simulink model "may7bdrc"  (Simulink 8.5)
settings: Solver=ode4  StartTime=0.0  StopTime=inf  FixedStep=BKIN_STEP_TIME  RelTol=1e-3
model workspace (MAT data in the model file):
  BARRIER_ROW = 5
  BKIN_KINEMATIC_FRAME_SIZE = 400
  BKIN_STEP_TIME = 0.00025
  CIRCLE_ROW = 2
  CIRCLE_STROKE = 10
  CIRCLE_STROKE_W = 11
  E_BARRIER_HIT = 6
  E_COLLISION_HIT = 7
  E_ENTER_PRESHOT_AREA = 2
  E_ENTER_START_AREA = 12
  E_EXIT = 13
  E_EXIT_PRESHOT_AREA = 10
  E_GOAL_HIT = 8
  E_GOAL_REACHED = 5
  E_NO_EVENT = 0
  E_PRESHOT_ROW = 4
  E_TARGET_OUT_OF_BOUNDS = 9
  E_TRIAL_BEGIN = 1
  E_TRIAL_ENDED = 3
  FIRST_STATE_FILL = 9
  FORCE_MULTIPLIER = 1
  F_BUMP = 1
  GOAL_ROW = 8
  GOAL_TIME = 15
  HEIGHT = 6
  INVISIBLE_FILL = 15
  LOAD_ROW = 4
  MASS_BARRIER = 6
  MASS_CIRCLE = 2
  MASS_RECT = 3
  NEW_FLOAT = 10
  NEW_ROW = 9
  NEW_TEXTSIZE = 11
  PERT_DUR = 5
  PERT_RAMP = 4
  PRESHOT_ROW = 7
  RADIUS_LOG = 4
  RADIUS_VIS = 5
  RECT_FILL = 12
  RECT_ROW = 3
  RECT_STROKE = 13
  RECT_STROKE_W = 14
  ROTATION = 7
  SECONDS = 1
  SECOND_STATE_FILL = 8
  SHOT_READY_TIME = 13
  SHOT_SET_TIME = 14
  START_HOLD_TIME = 12
  START_ROW = 6
  TRIAL_FAILURE = 11
  WIDTH = 3
  col_x = 1
  col_y = 2
StartFcn:
  |  warndlg('Dexterit-E models cannot run under simulation. Please compile your model and run it from within Dexterit-E.');set_param(bdroot,'SimulationCommand','stop')
undefined symbols (not defined in the file): slselsubs
libraries: Video x7, General x3, KINARM_loads x2, KINARM_EP_loads x1, KINARM_general x1, simulink x1, slrtlib x1
(part 1 of 3)
settings Model: Creator=Chris Grebeldinger  LastModifiedBy=User  ModifiedComment=chris -- Wed Feb 16 09:18:30 2005 -- Version 1.1384  ModifiedHistory=Feb 16/05 - Add error repeat, add offset ramp  ExtModeArmWhenConnect=off  ExtModeLogAll=off
settings SolverCC: AutoInsertRateTranBlk=on
settings DataIOCC: LimitDataPoints=off  SaveOutput=off  SaveTime=off  SignalLoggingName=sigsOut
settings OptimizationCC: BlockReduction=off  BooleanDataType=off  OptimizeBlockIOStorage=off  BufferReuse=off  GlobalBufferReuse=off  ExpressionFolding=off  LocalBlockOutputs=off  InitFltsAndDblsToZero=on
settings DebuggingCC: SaveWithParameterizedLinksMsg=none  SignalResolutionControl=TryResolveAllWithWarning  MultiTaskDSMMsg=warning  FcnCallInpInsideContextMsg=EnableAllAsWarning  BusObjectLabelMismatch=none  StrictBusMsg=ErrorOnBusTreatedAsVector
settings HardwareCC: ProdIntDivRoundTo=Zero  ProdEndianess=LittleEndian  ProdLongLongMode=on  ProdHWDeviceType=Generic->32-bit x86 compatible  TargetHWDeviceType=32-bit Generic
settings SFSimCC: SimParseCustomCode=off
settings RTWCC: Description=Simulink Real-Time  SystemTargetFile=slrt.tlc  TemplateMakefile=slrt_default_tmf  CodeExecutionProfiling=on  RTWCompilerOptimization=on
settings CodeAppCC: MaxIdLength=63
settings SimulinkRealTimeCC: TargetFcnLib=ansi_tfl_tmw.mat  GeneratePreprocessorConditionals=Disable all

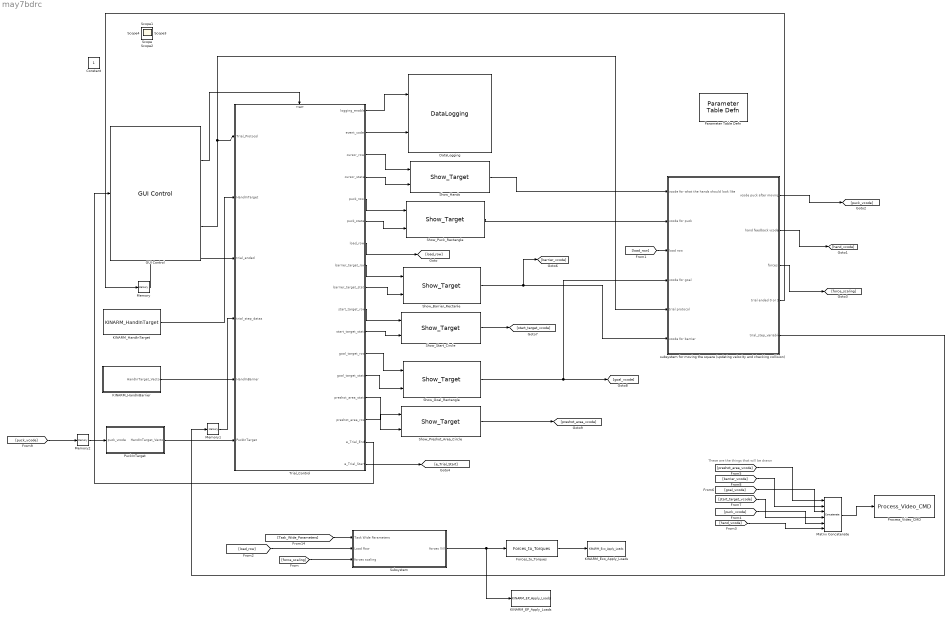
== system may7bdrc ==
  note: These are the things that will be drawn
  DataLogging : General/DataLogging  log_event_codes=on  log_analog_inputs=off  show_time_remaining=off  ecat_include=on
  Forces_to_Torques : KINARM_loads/Forces_to_Torques
  GUI Control : General/GUI Control  task_version=1.0  show_repeat_trial_flag=off  use_custom_tp=off  target_type_str=Circle  Target_Type=1  XYcols=[1 2]  Vcols=3  Lcols=4  indices_padding=[0 0 0 0;0 0 0 0]  target_table_rows=64  load_table_rows=20  tp_table_rows=100
  KINARM_EP_Apply_Loads : KINARM_EP_loads/KINARM_EP_Apply_Loads  up_duration=1500  down_duration=1500  max_force=20
  KINARM_Exo_Apply_Loads : KINARM_loads/KINARM_Exo_Apply_Loads  up_duration=1500  down_duration=1500  max_torque=5  limit_motors=off
  KINARM_HandInBarrier : Subsystem  AncestorBlock=KINARM_general/KINARM_HandInTarget  mask(KINARM_HandInTarget){use_dominant_hand=on, target_type=Rectangle, num_states=1, attribcol1=[WIDTH HEIGHT ROTATION], attribcol2=[0 0 0], attribcol3=[0 0 0], attribcol4=[0 0 0], attribcol5=[0 0 0]}
      mask prompts: use_dominant_hand "Use "arm to be assessed"?"; target_type "Type of Target"; num_states "Number of Target States"; attribcol1 "State 1 Target Table Column(s)"; attribcol2 "State 2 Target Table Column(s)"; attribcol3 "State 3 Target Table Column(s)"; attribcol4 "State 4 Target Table Column(s)"; attribcol5 "State 5 Target Table Column(s)"
      mask help: This block returns a vector or array corresponding to the Target_Table rows indicating whether the specified hand is in (=1) or out (=0) of each of the targets.
      mask init:
      | block_path = gcb;  % store block path, as gcb may change with block operations
      | 
      | %%% Get the model's workspace, because it is required to evaluate constants from the Parameter Table Def'n block
      | modelName=bdroot(block_path);
      | modelWorkspace = get_param(modelName, 'ModelWorkspace');
      | 
      | %%% Handle background colours if link status changes.  
      | checkBackgroundColour(block_path, 'KINARM_general');
      | 
      | %%% create the names of the input and output ports to display on the mask
      | % Select only the desired states for output. The output port is also renamed to reflect 
      | % whether the output is a vector (in the case of a single state) or an array (of vectors, 
      | % one for each of multiple states).
      | 
      | numStates = str2double( get_param(block_path, 'num_states') );
      | 
      | if numStates == 1
      | 	set_param([block_path '/Selected States'], 'Value', '[1]');
      | 	outputname = 'HandInTarget_Vector';
      | elseif numStates == 2
      | 	set_param([block_path '/Selected States'], 'Value', '[1,2]');
      | 	outputname = 'HandInTarget_Array';
      | elseif numStates == 3
      | 	set_param([block_path '/Selected States'], 'Value', '[1,2,3]');
      | 	outputname = 'HandInTarget_Array';
      | elseif numStates == 4
      | 	set_param([block_path '/Selected States'], 'Value', '[1,2,3,4]');
      | 	outputname = 'HandInTarget_Array';
      | else
      | 	set_param([block_path '/Selected States'], 'Value', '[1,2,3,4,5]');
      | 	outputname = 'HandInTarget_Array';
      | end
      | output_block=char(find_system(gcb,'LookUnderMasks','all','FollowLinks','on','SearchDepth',1,'BlockType','Outport'));
      | set_param(output_block, 'Name', outputname);
      | 
      | 
      | %%%%%%%%%%%%%%%%%%%%%%%%%%%%%%%%%%%%%%%%%%%%%%%%%%%%%%%%%%%%%
      | %%% Check and format the input strings for the vectors of column entires
      | targetTypeStr=get_param(block_path, 'target_type');
      | 
      | switch targetTypeStr(1:3)
      | 	case 'Cir',		numCol = 1;
      | 	case 'Ell',		numCol = 3;
      |     case 'Rec',		numCol = 3;
      |     case 'Lin',		numCol = 3;
      |     case 'Tri',		numCol = 4;
      | 	otherwise,		numCol = 1;
      | end
      | 
      | for ii = 1:numStates
      | 	variableName = ['attribcol' num2str(ii)];
      | 	attribcoltext = get_param(block_path, variableName);
      | 	attribcoltext = checkUserInputVectorLength(attribcoltext, numCol);
      | 	set_param(block_path, variableName, attribcoltext);
      | end
      | 
      | for ii = 1+numStates:5
      | 	variableName = ['attribcol' num2str(ii)];
      |     if numCol == 1
      |         outstr = '[0]';
      |     else
      |         outstr = mat2str(zeros(1, numCol));
      |     end
      |     set_param(block_path, variableName, outstr);
      | end
      | 
      | %%%%%%%%%%%%%%%%%%%%%%%%%%%%%%%%%%%%%%%%%%%%%%%%%%%%%%%%%%%%%
      | %%% Create the text to show on the mask
      | numStates = str2num(get_param(block_path, 'num_states'));
      | columntext='(columns: ';
      | 
      | for ii = 1:numStates
      | 	variableName = ['attribcol' num2str(ii)];
      | 	attribcolString = get_param(block_path, variableName);
      | 	if isempty(modelWorkspace)
      | 		% if the block is part of a library, then modelWorkspace will be empty and the other code to evaluate attribcolStringEval will fail
      | 		attribcolStringEval = '3';
      | 	else
      | 		[attribcolValue, errorMessage] = BKINevalin(modelWorkspace, attribcolString);
      | 		attribcolStringEval = mat2str( attribcolValue );
      | 	end
      | 	if ii > 1
      | 		columntext = [columntext, '; ', attribcolStringEval];
      | 	else
      | 		columntext = [columntext, attribcolStringEval];
      | 	end
      | end
      | 
      | % Add formatting spaces so that the mask looks nice
      | columntext=strvcat([columntext ')'],' ', ' ');
      mask Help:
      | Used to determine if the hand (fingertip) is in any of the targets in the Target_Table.
      | <P>
      | <B><I>Use of this block requires that the DataLogging block (General library) be set to log KINARM data.</I></B>
      | 
      | <H2>Library </H2>
      | KINARM general
      | 
      | <H2>Description </H2>
      | This block returns a vector or array corresponding to the Target_Table rows indicating whether the specified hand (i.e. fingertip) is in or out of each of the targets.  Each element in the output vector or output array will be either a 0 (hand not in target) or a 1 (hand in target).
      | <P>
      | A vector is returned if only one target state is specified in each target row (see Parameters and Dialog Box), with each index of the vector corresponding to a row in the target table.  An array is returned if more than one target state is specified in a target row, with each row of the array corresponding to a target row and each column corresponding to the nth target state specified in each target row.
      | <P>
      | The output vector or array is typically used by a stateflow chart to affect behavior of the system.  Because this block returns hand-in-target information for all targets in the target table, multiple targets can be monitored at once (i.e. the Stateflow chart could have certain transitions that occur if the hand is in one target and other transitions if it is in a different target).  Likewise, because this block returns hand-in-target information for multiple states of a single target, those multiple states can be monitored simultaneously.
      | <P>
      | Because the KINARM_HandInTarget block returns information for only one hand, two copies of this block are required if information for both hands is desired.
      | <P>
      | 
      | <H2>Parameters and Dialog Box</H2>
      | <B>Use "arm to be assessed"?:</B> this checkbox determines which hand is used by this block. In Dexterit-E the operator selects the "arm to be assessed" using radio buttons.
      | When this box is checked the output of this block is derived from the hand information corresponding to the arm selection made by the operator in Dexterit-E.
      | When this box is unchecked the output of this block is derived from the contralateral arm.
      | (Note: to obtain information about both hands, then 2 separate copies of this block are required - one for each hand.)
      | <P>
      | <B>Type of Target:</B> Enter the type of target specified in the target table:
      | <P>
      | <B>Number of Target States:</B> Enter the number of target states specified in each target row.  Up to four target states are allowed per target row.
      | <P>
      | <B>State <n> Target Table Columns:</B> Enter the columns in the Target Table that specify the relevant target attributes.  Do this for each target state.
      | For a circle, enter the columns corresponding to logical radius (e.g. 4)
      | <BR>For an ellipse, enter the columns corresponding to major radius, minor radius, rotation angle (e.g. [4, 5, 6]).
      | <BR>For a rectangle, enter the columns corresponding to length, height, and rotation angle (e.g. [4, 5, 6]).
      | <BR>For a line, enter the columns corresponding to stroke width, endpoint in x, and endpoint in y (e.g. [3, 4, 5]).
      | <BR>For a triangle, enter the columns corresponding to length, height, peak offset, and rotation angle (e.g. [4, 5, 6, 7]).
      | 
      | <H2>Examples</H2>
      | <B>Example 1.</B>  Suppose a target row will be used to define 1 state for a circle type target and the radius of the visual target is the same radius to be used for determination of hand-in-target.  The related Target Table column is: column 6 = radius.  For this example, "State 1 Target Table Columns" would equal [6].
      | <P>
      | 
      | <B>Example 2.</B>  Suppose a target row will be used to define 1 state for a circle type target, but the radius of the visual target will be different than the radius to be used for determination of hand-in-target.  This option allows independent control over the size of the visual target versus the accuracy needed to be considered "in the target".  The related Target Table columns are: column 6 = radius1 (i.e. radius to target to be drawn); column 7 = radius2 (i.e. radius to be used for hand-in-target) .  For this example, "State 1 Target Table Columns" would equal [7].
      | <P>
      | <B>Example 3.</B>  Suppose a target row will be used to define 2 states for a circle type target, where the radius of the visual target will be a constant, but depending on the state of the system, one of 2 other and different radii will be used for determination of hand-in-target.  The related Target Table columns are: column 6 = radius1 (i.e. radius to target to be drawn); column 7 = radius2 (i.e. radius to be used for hand-in-target for state 1); column 8 = radius3 (i.e. radius to be used for hand-in-target for state 2).  For this example, "State 1 Target Table Columns" would equal [7], while "State 2 Target Table Columns" would equal [8].
      | <P>
      | 
      | <H2>Related Blocks </H2>
      | DataLogging
      mask TypeOptions target_type: Circle | Ellipse | Rectangle | Line | Triangle
      mask Callback target_type:
      | %%%%
      | % Because of bugs iN R2007, R2010a and R2013a (which have been reported to Mathworks), the following code
      | % is required here because in the Initialization Section it will ONLY correctly update those Mask Parameters that are hidden
      | % when the OK button is clicked (NOTE: the initialization code will correctly update all Mask Parameters when the Apply button
      | % is clicked, the bug is that it should also update everything when the OK button is clicked in the absence of an Apply click)
      | %
      | % Adding a set_param call which updates one of the mask parameters will call the initialization code to run, which "avoids"
      | % this bug. This code should be removed once Mathworks has fixed this bug.
      | 
      | temp = get_param(gcb, 'target_type');
      | set_param(gcb, 'target_type', temp);
      mask TypeOptions num_states: 1 | 2 | 3 | 4 | 5
      mask Callback num_states:
      | num_states = str2num(get_param(gcb, 'num_states'));
      | vis = get_param(gcb, 'MaskVisibilities');
      | 
      | % Select only the desired states for output. The output port is also renamed to reflect
      | % whether the output is a vector (in the case of a single state) or an array (of vectors,
      | % one for each of multiple states).
      | output_block=char(find_system(gcb, 'LookUnderMasks', 'all', 'FollowLinks', 'on', 'SearchDepth', 1, 'BlockType', 'Outport'));
      | 
      | if num_states == 1
      | % % % 	set_param([gcb '/Selected States'], 'Value', '[1]');
      | % % % 	set_param(output_block, 'Name', 'HandInTarget_Vector');
      | 	vis{5} = 'off';
      | 	vis{6} = 'off';
      | 	vis{7} = 'off';
      | 	vis{8} = 'off';
      | elseif num_states == 2
      | % % % 	set_param([gcb '/Selected States'], 'Value', '[1,2]');
      | % % % 	set_param(output_block, 'Name', 'HandInTarget_Array');
      | 	vis{5} = 'on';
      | 	vis{6} = 'off';
      | 	vis{7} = 'off';
      | 	vis{8} = 'off';
      | elseif num_states == 3
      | % % % 	set_param([gcb '/Selected States'], 'Value', '[1,2,3]');
      | % % % 	set_param(output_block, 'Name','HandInTarget_Array');
      | 	vis{5} = 'on';
      | 	vis{6} = 'on';
      | 	vis{7} = 'off';
      | 	vis{8} = 'off';
      | elseif num_states == 4
      | % % % 	set_param([gcb '/Selected States'], 'Value', '[1,2,3,4]');
      | % % % 	set_param(output_block, 'Name','HandInTarget_Array');
      | 	vis{5} = 'on';
      | 	vis{6} = 'on';
      | 	vis{7} = 'on';
      | 	vis{8} = 'off';
      | else
      | % % % 	set_param([gcb '/Selected States'], 'Value', '[1,2,3,4,5]');
      | % % % 	set_param(output_block, 'Name', 'HandInTarget_Array');
      | 	vis{5} = 'on';
      | 	vis{6} = 'on';
      | 	vis{7} = 'on';
      | 	vis{8} = 'on';
      | end
      | set_param(gcb, 'MaskVisibilities', vis);
      mask Display:
      | disp(columntext);
      | port_label('output',1,outputname);
  KINARM_HandInTarget : KINARM_general/KINARM_HandInTarget  use_dominant_hand=on  target_type=Circle  num_states=1  attribcol1=[RADIUS_LOG]  attribcol2=[0]  attribcol3=[0]  attribcol4=[0]  attribcol5=[0]
  Matrix Concatenate : Concatenate  NumInputs=6  Mode=Multidimensional array
  Memory : Memory
  Memory1 : Memory
  Memory2 : Memory
  Parameter Table Defn : General/Parameter Table Defn  ShowInLibBrowser=0
  Process_Video_CMD : Video/Process_Video_CMD  video_delay=0
  PuckInTarget : Subsystem  AncestorBlock=KINARM_general/KINARM_HandInTarget  mask(KINARM_HandInTarget){use_dominant_hand=on, target_type=Rectangle, num_states=1, attribcol1=[WIDTH HEIGHT ROTATION], attribcol2=[0 0 0], attribcol3=[0 0 0], attribcol4=[0 0 0], attribcol5=[0 0 0]}
      mask prompts: use_dominant_hand "Use "arm to be assessed"?"; target_type "Type of Target"; num_states "Number of Target States"; attribcol1 "State 1 Target Table Column(s)"; attribcol2 "State 2 Target Table Column(s)"; attribcol3 "State 3 Target Table Column(s)"; attribcol4 "State 4 Target Table Column(s)"; attribcol5 "State 5 Target Table Column(s)"
      mask help: This block returns a vector or array corresponding to the Target_Table rows indicating whether the specified hand is in (=1) or out (=0) of each of the targets.
      mask init: same as may7bdrc/KINARM_HandInBarrier
      mask Help:
      | Used to determine if the hand (fingertip) is in any of the targets in the Target_Table.
      | <P>
      | <B><I>Use of this block requires that the DataLogging block (General library) be set to log KINARM data.</I></B>
      | 
      | <H2>Library </H2>
      | KINARM general
      | 
      | <H2>Description </H2>
      | This block returns a vector or array corresponding to the Target_Table rows indicating whether the specified hand (i.e. fingertip) is in or out of each of the targets.  Each element in the output vector or output array will be either a 0 (hand not in target) or a 1 (hand in target).
      | <P>
      | A vector is returned if only one target state is specified in each target row (see Parameters and Dialog Box), with each index of the vector corresponding to a row in the target table.  An array is returned if more than one target state is specified in a target row, with each row of the array corresponding to a target row and each column corresponding to the nth target state specified in each target row.
      | <P>
      | The output vector or array is typically used by a stateflow chart to affect behavior of the system.  Because this block returns hand-in-target information for all targets in the target table, multiple targets can be monitored at once (i.e. the Stateflow chart could have certain transitions that occur if the hand is in one target and other transitions if it is in a different target).  Likewise, because this block returns hand-in-target information for multiple states of a single target, those multiple states can be monitored simultaneously.
      | <P>
      | Because the KINARM_HandInTarget block returns information for only one hand, two copies of this block are required if information for both hands is desired.
      | <P>
      | 
      | <H2>Parameters and Dialog Box</H2>
      | <B>Use "arm to be assessed"?:</B> this checkbox determines which hand is used by this block. In Dexterit-E the operator selects the "arm to be assessed" using radio buttons.
      | When this box is checked the output of this block is derived from the hand information corresponding to the arm selection made by the operator in Dexterit-E.
      | When this box is unchecked the output of this block is derived from the contralateral arm.
      | (Note: to obtain information about both hands, then 2 separate copies of this block are required - one for each hand.)
      | <P>
      | <B>Type of Target:</B> Enter the type of target specified in the target table:
      | <P>
      | <B>Number of Target States:</B> Enter the number of target states specified in each target row.  Up to four target states are allowed per target row.
      | <P>
      | <B>State <n> Target Table Columns:</B> Enter the columns in the Target Table that specify the relevant target attributes.  Do this for each target state.
      | For a circle, enter the columns corresponding to logical radius (e.g. 4)
      | <BR>For an ellipse, enter the columns corresponding to major radius, minor radius, rotation angle (e.g. [4, 5, 6]).
      | <BR>For a rectangle, enter the columns corresponding to length, height, and rotation angle (e.g. [4, 5, 6]).
      | <BR>For a line, enter the columns corresponding to stroke width, endpoint in x, and endpoint in y (e.g. [3, 4, 5]).
      | <BR>For a triangle, enter the columns corresponding to length, height, peak offset, and rotation angle (e.g. [4, 5, 6, 7]).
      | 
      | <H2>Examples</H2>
      | <B>Example 1.</B>  Suppose a target row will be used to define 1 state for a circle type target and the radius of the visual target is the same radius to be used for determination of hand-in-target.  The related Target Table column is: column 6 = radius.  For this example, "State 1 Target Table Columns" would equal [6].
      | <P>
      | 
      | <B>Example 2.</B>  Suppose a target row will be used to define 1 state for a circle type target, but the radius of the visual target will be different than the radius to be used for determination of hand-in-target.  This option allows independent control over the size of the visual target versus the accuracy needed to be considered "in the target".  The related Target Table columns are: column 6 = radius1 (i.e. radius to target to be drawn); column 7 = radius2 (i.e. radius to be used for hand-in-target) .  For this example, "State 1 Target Table Columns" would equal [7].
      | <P>
      | <B>Example 3.</B>  Suppose a target row will be used to define 2 states for a circle type target, where the radius of the visual target will be a constant, but depending on the state of the system, one of 2 other and different radii will be used for determination of hand-in-target.  The related Target Table columns are: column 6 = radius1 (i.e. radius to target to be drawn); column 7 = radius2 (i.e. radius to be used for hand-in-target for state 1); column 8 = radius3 (i.e. radius to be used for hand-in-target for state 2).  For this example, "State 1 Target Table Columns" would equal [7], while "State 2 Target Table Columns" would equal [8].
      | <P>
      | 
      | <H2>Related Blocks </H2>
      | DataLogging
      mask TypeOptions target_type: Circle | Ellipse | Rectangle | Line | Triangle
      mask Callback target_type:
      | %%%%
      | % Because of bugs iN R2007, R2010a and R2013a (which have been reported to Mathworks), the following code
      | % is required here because in the Initialization Section it will ONLY correctly update those Mask Parameters that are hidden
      | % when the OK button is clicked (NOTE: the initialization code will correctly update all Mask Parameters when the Apply button
      | % is clicked, the bug is that it should also update everything when the OK button is clicked in the absence of an Apply click)
      | %
      | % Adding a set_param call which updates one of the mask parameters will call the initialization code to run, which "avoids"
      | % this bug. This code should be removed once Mathworks has fixed this bug.
      | 
      | temp = get_param(gcb, 'target_type');
      | set_param(gcb, 'target_type', temp);
      mask TypeOptions num_states: 1 | 2 | 3 | 4 | 5
      mask Callback num_states:
      | num_states = str2num(get_param(gcb, 'num_states'));
      | vis = get_param(gcb, 'MaskVisibilities');
      | 
      | % Select only the desired states for output. The output port is also renamed to reflect
      | % whether the output is a vector (in the case of a single state) or an array (of vectors,
      | % one for each of multiple states).
      | output_block=char(find_system(gcb, 'LookUnderMasks', 'all', 'FollowLinks', 'on', 'SearchDepth', 1, 'BlockType', 'Outport'));
      | 
      | if num_states == 1
      | % % % 	set_param([gcb '/Selected States'], 'Value', '[1]');
      | % % % 	set_param(output_block, 'Name', 'HandInTarget_Vector');
      | 	vis{5} = 'off';
      | 	vis{6} = 'off';
      | 	vis{7} = 'off';
      | 	vis{8} = 'off';
      | elseif num_states == 2
      | % % % 	set_param([gcb '/Selected States'], 'Value', '[1,2]');
      | % % % 	set_param(output_block, 'Name', 'HandInTarget_Array');
      | 	vis{5} = 'on';
      | 	vis{6} = 'off';
      | 	vis{7} = 'off';
      | 	vis{8} = 'off';
      | elseif num_states == 3
      | % % % 	set_param([gcb '/Selected States'], 'Value', '[1,2,3]');
      | % % % 	set_param(output_block, 'Name','HandInTarget_Array');
      | 	vis{5} = 'on';
      | 	vis{6} = 'on';
      | 	vis{7} = 'off';
      | 	vis{8} = 'off';
      | elseif num_states == 4
      | % % % 	set_param([gcb '/Selected States'], 'Value', '[1,2,3,4]');
      | % % % 	set_param(output_block, 'Name','HandInTarget_Array');
      | 	vis{5} = 'on';
      | 	vis{6} = 'on';
      | 	vis{7} = 'on';
      | 	vis{8} = 'off';
      | else
      | % % % 	set_param([gcb '/Selected States'], 'Value', '[1,2,3,4,5]');
      | % % % 	set_param(output_block, 'Name', 'HandInTarget_Array');
      | 	vis{5} = 'on';
      | 	vis{6} = 'on';
      | 	vis{7} = 'on';
      | 	vis{8} = 'on';
      | end
      | set_param(gcb, 'MaskVisibilities', vis);
      mask Display:
      | disp(columntext);
      | port_label('output',1,outputname);
  Show_Barrier_Rectanle : Video/Show_Target  target_type=Rectangle  num_states=2  attribcol1=[FIRST_STATE_FILL RECT_STROKE RECT_STROKE_W WIDTH HEIGHT ROTATION]  attribcol2=[SECOND_STATE_FILL RECT_STROKE RECT_STROKE_W WIDTH HEIGHT ROTATION]  attribcol3=[0 0 0 0 0 0]  attribcol4=[0 0 0 0 0 0]  attribcol5=[0 0 0 0 0 0]  stateindices_padding=[0 0 0 0 0;0 0 0 0 0;0 0 0 0 0;0 0 0 0 0;0 0 0 0 0]  source=dialog  opacity=100  target_display=Both subject and operator displays  num_col=6
  Show_Goal_Rectangle : Video/Show_Target  target_type=Rectangle  num_states=3  attribcol1=[INVISIBLE_FILL RECT_STROKE RECT_STROKE_W WIDTH HEIGHT ROTATION]  attribcol2=[FIRST_STATE_FILL RECT_STROKE RECT_STROKE_W WIDTH HEIGHT ROTATION]  attribcol3=[SECOND_STATE_FILL RECT_STROKE RECT_STROKE_W WIDTH HEIGHT ROTATION]  attribcol4=[0 0 0 0 0 0]  attribcol5=[0 0 0 0 0 0]  stateindices_padding=[0 0 0 0 0;0 0 0 0 0;0 0 0 0 0;0 0 0 0 0;0 0 0 0 0]  source=dialog  opacity=100  target_display=Both subject and operator displays  num_col=6
  Show_Hands : Video/Show_Target  target_type=Circle  num_states=2  attribcol1=[FIRST_STATE_FILL CIRCLE_STROKE CIRCLE_STROKE_W WIDTH]  attribcol2=[SECOND_STATE_FILL CIRCLE_STROKE CIRCLE_STROKE_W WIDTH]  attribcol3=[0 0 0 0]  attribcol4=[0 0 0 0]  attribcol5=[0 0 0 0]  stateindices_padding=[0 0 0 0 0 0 0;0 0 0 0 0 0 0;0 0 0 0 0 0 0;0 0 0 0 0 0 0;0 0 0 0 0 0 0]  source=dialog  opacity=100  target_display=Both subject and operator displays  num_col=4
  Show_Preshot_Area_Circle : Video/Show_Target  target_type=Circle  num_states=3  attribcol1=[INVISIBLE_FILL CIRCLE_STROKE CIRCLE_STROKE_W WIDTH]  attribcol2=[FIRST_STATE_FILL CIRCLE_STROKE CIRCLE_STROKE_W WIDTH]  attribcol3=[SECOND_STATE_FILL CIRCLE_STROKE CIRCLE_STROKE_W WIDTH]  attribcol4=[0 0 0 0]  attribcol5=[0 0 0 0]  stateindices_padding=[0 0 0 0 0 0 0;0 0 0 0 0 0 0;0 0 0 0 0 0 0;0 0 0 0 0 0 0;0 0 0 0 0 0 0]  source=dialog  opacity=100  target_display=Both subject and operator displays  num_col=4
  Show_Puck_Rectangle : Video/Show_Target  target_type=Rectangle  num_states=3  attribcol1=[INVISIBLE_FILL RECT_STROKE RECT_STROKE_W WIDTH HEIGHT ROTATION]  attribcol2=[FIRST_STATE_FILL RECT_STROKE RECT_STROKE_W WIDTH HEIGHT ROTATION]  attribcol3=[SECOND_STATE_FILL RECT_STROKE RECT_STROKE_W WIDTH HEIGHT ROTATION]  attribcol4=[0 0 0 0 0 0]  attribcol5=[0 0 0 0 0 0]  stateindices_padding=[0 0 0 0 0;0 0 0 0 0;0 0 0 0 0;0 0 0 0 0;0 0 0 0 0]  source=dialog  opacity=100  target_display=Both subject and operator displays  num_col=6
  Show_Start_Circle : Video/Show_Target  target_type=Circle  num_states=3  attribcol1=[INVISIBLE_FILL CIRCLE_STROKE CIRCLE_STROKE_W WIDTH]  attribcol2=[FIRST_STATE_FILL CIRCLE_STROKE CIRCLE_STROKE_W WIDTH]  attribcol3=[SECOND_STATE_FILL CIRCLE_STROKE CIRCLE_STROKE_W WIDTH]  attribcol4=[0 0 0 0]  attribcol5=[0 0 0 0]  stateindices_padding=[0 0 0 0 0 0 0;0 0 0 0 0 0 0;0 0 0 0 0 0 0;0 0 0 0 0 0 0;0 0 0 0 0 0 0]  source=dialog  opacity=100  target_display=Both subject and operator displays  num_col=4
  Subsystem : Subsystem
  Trial_Control : Stateflow chart  TreatAsAtomicUnit=on
      settings: PermitHierarchicalResolution=ParametersOnly
  subsystem for moving the square (updating velocity and checking collision) : Subsystem
  Constant : Constant  IOType=siggen
  Scope{,1..4} (5 alike) : Scope
      Scope settings: TimeRange=auto  MaxDataPoints=5000  SaveToWorkspace=off  SaveName=ScopeData  YMin=-10.00000  YMax=10.00000  SampleTime=-1
      Scope1 settings: TimeRange=auto  MaxDataPoints=5000  SaveToWorkspace=off  YMin=-10.00000  YMax=10.00000  SampleTime=-1
      Scope2 settings: TimeRange=auto  MaxDataPoints=5000  SaveToWorkspace=off  SaveName=ScopeData2  YMin=-10.00000  YMax=10.00000  SampleTime=-1
      Scope3 settings: TimeRange=auto  MaxDataPoints=5000  SaveToWorkspace=off  SaveName=ScopeData3  YMin=-10.00000  YMax=10.00000  SampleTime=-1
      Scope4 settings: TimeRange=auto  MaxDataPoints=5000  SaveToWorkspace=off  SaveName=ScopeData4  YMin=-10.00000  YMax=10.00000  SampleTime=-1
  wires:
  Trial_Control/3(cursor_row) -> Show_Hands/1
  Trial_Control/5(puck_row) -> Show_Puck_Rectangle/1
  Trial_Control/6(puck_state) -> Show_Puck_Rectangle/2
  Forces_to_Torques/1 -> KINARM_Exo_Apply_Loads/1
  Trial_Control/1(logging_enable) -> DataLogging/1
  Trial_Control/7(load_row) -> [load_row]
  Trial_Control/16(e_Trial_End) -> GUI Control/1
  Trial_Control/4(cursor_state) -> Show_Hands/2
  GUI Control/1 -> Trial_Control/Trigger
  Matrix Concatenate/1 -> Process_Video_CMD/1
  Show_Hands/1 -> subsystem for moving the square (updating velocity and checking collision)/1(vcode for what the hands should look like)
  Show_Puck_Rectangle/1 -> subsystem for moving the square (updating velocity and checking collision)/2(vcode for puck)
  subsystem for moving the square (updating velocity and checking collision)/1(vcode puck after moving) -> [puck_vcode]
  subsystem for moving the square (updating velocity and checking collision)/3(forces) -> [force_scaling]
  subsystem for moving the square (updating velocity and checking collision)/2(hand feedback vcode) -> [hand_vcode]
  Trial_Control/2(event_code) -> DataLogging/2
  Subsystem/1(forces (N)) -> KINARM_EP_Apply_Loads/1, Forces_to_Torques/1
  [Task_Wide_Parameters] -> Subsystem/1(Task Wide Parameters)
  [load_row] -> Subsystem/2(Load Row)
  [force_scaling] -> Subsystem/3(forces scaling)
  [load_row] -> subsystem for moving the square (updating velocity and checking collision)/3(load row)
  Trial_Control/8(barrier_target_row) -> Show_Barrier_Rectanle/1
  Trial_Control/9(barrier_target_state) -> Show_Barrier_Rectanle/2
  Trial_Control/10(start_target_row) -> Show_Start_Circle/1
  Trial_Control/11(start_target_state) -> Show_Start_Circle/2
  Trial_Control/12(goal_target_row) -> Show_Goal_Rectangle/1
  Trial_Control/13(goal_target_state) -> Show_Goal_Rectangle/2
  KINARM_HandInTarget/1 -> Trial_Control/2(HandInTarget)
  GUI Control/2 -> subsystem for moving the square (updating velocity and checking collision)/5(trial protocol), Trial_Control/1(Trial_Protocol)
  subsystem for moving the square (updating velocity and checking collision)/4(trial ended 0 or 1) -> Memory/1
  Memory/1 -> Trial_Control/3(trial_ended)
  subsystem for moving the square (updating velocity and checking collision)/5(trial_step_variable) -> Memory1/1
  Memory1/1 -> Trial_Control/4(trial_step_datas)
  Show_Barrier_Rectanle/1 -> [barrier_vcode], subsystem for moving the square (updating velocity and checking collision)/6(vcode for barrier)
  Show_Preshot_Area_Circle/1 -> [preshot_area_vcode]
  Show_Goal_Rectangle/1 -> subsystem for moving the square (updating velocity and checking collision)/4(vcode for goal), [goal_vcode]
  Show_Start_Circle/1 -> [start_target_vcode]
  Trial_Control/14(preshot_area_state) -> Show_Preshot_Area_Circle/2
  Trial_Control/15(preshot_area_row) -> Show_Preshot_Area_Circle/1
  [hand_vcode] -> Matrix Concatenate/6
  [puck_vcode] -> Matrix Concatenate/5
  [preshot_area_vcode] -> Matrix Concatenate/1
  [barrier_vcode] -> Matrix Concatenate/2
  [goal_vcode] -> Matrix Concatenate/3
  [start_target_vcode] -> Matrix Concatenate/4
  KINARM_HandInBarrier/1(HandInTarget_Vector) -> Trial_Control/5(HandInBarrier)
  [puck_vcode] -> Memory2/1
  PuckInTarget/1(HandInTarget_Vector) -> Trial_Control/6(PuckInTarget)
  Memory2/1 -> PuckInTarget/1(puck_vcode)
  Trial_Control/17(e_Trial_Start) -> [e_Trial_Start]

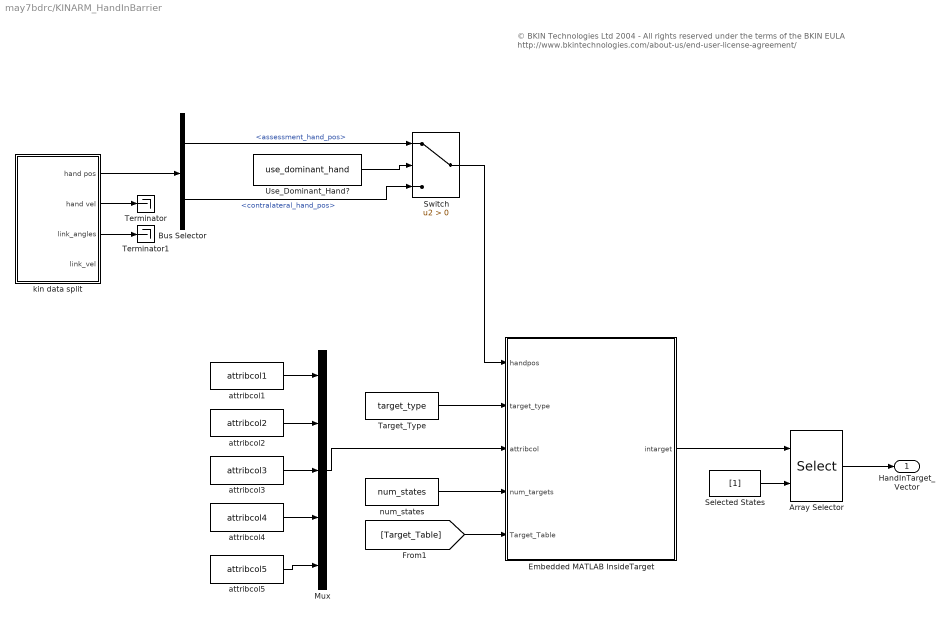
== system may7bdrc/KINARM_HandInBarrier ==
  note: © BKIN Technologies Ltd 2004  - All rights reserved under the terms of the BKIN EULA
      | http://www.bkintechnologies.com/about-us/end-user-license-agreement/
  Array Selector : Selector  NumberOfDimensions=2  InputPortWidth=3  IndexOptions=Select all,Index vector (port)  Indices=-1,1  OutputSizes=slselsubs([(-2),(-2)],1),slselsubs([(-2),(-2)],2)
  Bus Selector : BusSelector  OutputSignals=assessment_hand_pos,contralateral_hand_pos
  Embedded MATLAB InsideTarget : MATLAB Function  TreatAsAtomicUnit=on
      settings: PermitHierarchicalResolution=ParametersOnly  RTWSystemCode=Nonreusable function  RTWFileNameOpts=Use function name
  Mux : Mux  Inputs=5
  Selected States : Constant  Value=[1]
  Switch : Switch  Criteria=u2 > Threshold
  Target_Type : Constant  Value=target_type
  Terminator : Terminator
  Terminator1 : Terminator
  Use_Dominant_Hand? : Constant  Value=use_dominant_hand
  attribcol1 : Constant  Value=attribcol1
  attribcol2 : Constant  Value=attribcol2
  attribcol3 : Constant  Value=attribcol3
  attribcol4 : Constant  Value=attribcol4
  attribcol5 : Constant  Value=attribcol5
  kin data split : Subsystem
  num_states : Constant  Value=num_states
  HandInTarget_Vector : Outport
  wires:
  Selected States/1 -> Array Selector/2
  num_states/1 -> Embedded MATLAB InsideTarget/4(num_targets)
  Mux/1 -> Embedded MATLAB InsideTarget/3(attribcol)
  attribcol4/1 -> Mux/4
  attribcol3/1 -> Mux/3
  attribcol2/1 -> Mux/2
  attribcol1/1 -> Mux/1
  Target_Type/1 -> Embedded MATLAB InsideTarget/2(target_type)
  Array Selector/1 -> HandInTarget_Vector/1
  [Target_Table] -> Embedded MATLAB InsideTarget/5(Target_Table)
  Embedded MATLAB InsideTarget/1(intarget) -> Array Selector/1
  attribcol5/1 -> Mux/5
  kin data split/1(hand pos) -> Bus Selector/1
  Use_Dominant_Hand?/1 -> Switch/2
  Bus Selector/1 -> Switch/1  "<assessment_hand_pos>"
  Bus Selector/2 -> Switch/3  "<contralateral_hand_pos>"
  kin data split/2(hand vel) -> Terminator/1
  kin data split/3(link_angles) -> Terminator1/1
  Switch/1 -> Embedded MATLAB InsideTarget/1(handpos)

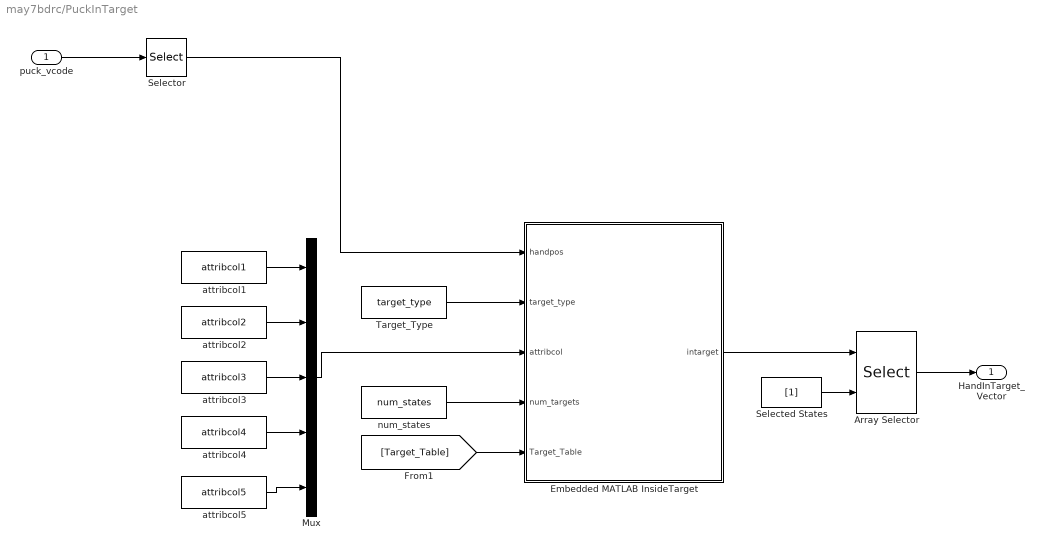
== system may7bdrc/PuckInTarget ==
  puck_vcode : Inport  PortDimensions=[1,70]
  Array Selector : Selector  NumberOfDimensions=2  InputPortWidth=3  IndexOptions=Select all,Index vector (port)  Indices=-1,1  OutputSizes=slselsubs([(-2),(-2)],1),slselsubs([(-2),(-2)],2)
  Embedded MATLAB InsideTarget : MATLAB Function  TreatAsAtomicUnit=on
      settings: PermitHierarchicalResolution=ParametersOnly  RTWSystemCode=Nonreusable function  RTWFileNameOpts=Use function name
  Mux : Mux  Inputs=5
  Selected States : Constant  Value=[1]
  Selector : Selector  NumberOfDimensions=2  InputPortWidth=3  IndexOptions=Index vector (dialog),Index vector (dialog)  Indices=1,[3,4]  OutputSizes=1,1
  Target_Type : Constant  Value=target_type
  attribcol1 : Constant  Value=attribcol1
  attribcol2 : Constant  Value=attribcol2
  attribcol3 : Constant  Value=attribcol3
  attribcol4 : Constant  Value=attribcol4
  attribcol5 : Constant  Value=attribcol5
  num_states : Constant  Value=num_states
  HandInTarget_Vector : Outport
  wires:
  Selected States/1 -> Array Selector/2
  num_states/1 -> Embedded MATLAB InsideTarget/4(num_targets)
  Mux/1 -> Embedded MATLAB InsideTarget/3(attribcol)
  attribcol4/1 -> Mux/4
  attribcol3/1 -> Mux/3
  attribcol2/1 -> Mux/2
  attribcol1/1 -> Mux/1
  Target_Type/1 -> Embedded MATLAB InsideTarget/2(target_type)
  Array Selector/1 -> HandInTarget_Vector/1
  [Target_Table] -> Embedded MATLAB InsideTarget/5(Target_Table)
  Embedded MATLAB InsideTarget/1(intarget) -> Array Selector/1
  attribcol5/1 -> Mux/5
  Selector/1 -> Embedded MATLAB InsideTarget/1(handpos)
  puck_vcode/1 -> Selector/1

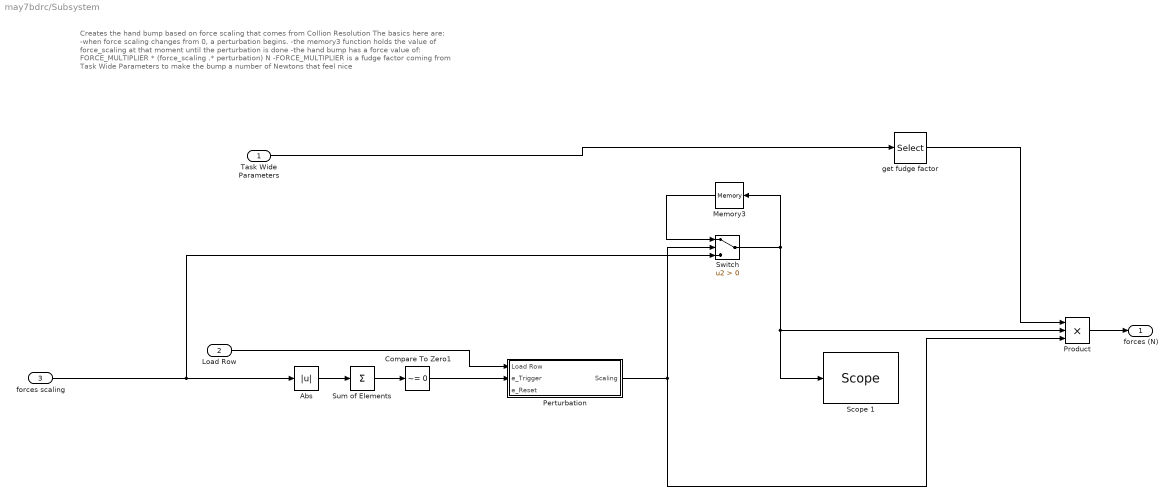
== system may7bdrc/Subsystem ==
  note: Creates the hand bump based on force scaling that comes from Collion Resolution
      |
      | The basics here are:
      | -when force scaling changes from 0, a perturbation begins.
      | -the memory3 function holds the value of force_scaling at that moment until the perturbation is done
      | -the hand bump has a force value of: FORCE_MULTIPLIER * (force_scaling .* perturbation) N
      | -FORCE_MULTIPLIER is a fudge factor coming from Task Wide Parameters to make the bump a number of Newtons that feel nice
  Task Wide Parameters : Inport
  Load Row : Inport  Port=2
  forces scaling : Inport  Port=3
  Abs : Abs
  Compare To Zero1 : simulink/Logic and Bit Operations/Compare To Zero  relop=~=  OutDataTypeStr=uint8  ZeroCross=off
  Memory3 : Memory  InheritSampleTime=on
  Perturbation : Subsystem  AncestorBlock=KINARM_loads/Perturbation  mask(Perturbation){loadcol=[PERT_RAMP PERT_DUR PERT_RAMP]}
      mask prompts: loadcol "Load Table Columns [colA colB colC]"
      mask help:
      | The Perturbation block creates a time-varying output that is used to ‘window’ the output of other load  blocks.  For example, to create a force pulse, the 'scaling' output of this block would be wired into the 'scaling' input of the Constant_Loads_(hand) block.
      |
      | The shape of the scaling window is trapezoidal and composed of three sections:
      |
      | 1. A linear on-ramp where the scaling output goes from 0 to 1. The duration of this ramping is determined from the value in column A.
      | 2. A duration where the scaling output is 1 (i.e. maximal). This duration is determined from the value in column B.
      | 3. A linear off-ramp where the scaling output goes from 1 to 0. The duration of this ramping is determined from the value in column C.
      |
      | (Note: scaling output = 0 between perturbations)
      |
      | The values in columns A, B & C must all be in milliseconds.
      |
      | The reset input is used to immediately stop the perturbation and set the output scaling to zero. The reset input does not need to be called between uses.
      mask init:
      | library = 'KINARM_loads';
      | numCol = 3;
      | [inputname1, inputname2, inputname3, outputname, columntext] = loadBlockInitCommands(gcb, library, numCol);
      mask Help:
      | Used to create a perturbation 'window' for scaling other load blocks.
      | 
      | <H2>Library </H2>
      | KINARM EXO loads
      | 
      | <H2>Description </H2>
      | The Perturbation block creates a time-varying output that is used to ‘window’ the output of other load blocks.  The 'scaling' output of the Perturbation block is typically wired to the 'scaling' input of another load block (note: the 'scaling' input of other loads blocks is hidden by default and must be shown by setting the 'Source for scaling' to 'external' within that block’s dialog box).
      | <P>
      | <P>
      | The perturbation window is started by sending a Stateflow event to the trigger input.  Once the perturbation has started, it continues in a deterministic fashion to its end unless a Stateflow event is sent to the 'reset' input, in which case the perturbation is canceled and the 'scaling' output is set to 0.
      | 
      | <p>The shape of the scaling window is trapezoidal and composed of three sections:
      | 
      | <ol>
      | <li>A linear on-ramp where the scaling output goes from 0 to 1. The duration of this ramping is determined from the value in column A.</li>
      | <li>A duration where the scaling output is 1 (i.e. maximal). This duration is determined from the value in column B.</li>
      | <li>A linear off-ramp where the scaling output goes from 1 to 0. The duration of this ramping is determined from the value in column C.</li>
      | </ol>
      | 
      | The ramp duration parameters [A, B, C] are found in the Load Table using the 'row' input to this block and the 'columns' parameter found in the dialog box for this block.
      | <p>For example, if the "row" input = 2, and "Load Table columns" are specified as [1 2 3], then using the sample Load Table below, the duration of the on ramp is 100 ms, constant torque is 200 ms, and the off ramp is 500 ms.
      | <br>
      | (Note: scaling output = 0 between perturbations)
      | 
      | <table border="1" cellpadding="5">
      | <tr><td></td><td>Ramp On</td><td>Const</td><td>Ramp off</td></tr>
      | <tr><td>Load 1</td><td>25</td><td>25</td><td>25</td></tr>
      | <tr><td>Load 2</td><td>100</td><td>200</td><td>500</td></tr>
      | <tr><td>Load 3</td><td>25</td><td>50</td><td>75</td></tr>
      | </table>
      | <P>
      | <B>row: </B> this scalar input indicates which row in the Load Table the ramp duration parameters [A, B, C] will come from.
      | <P>
      | <B>trigger: </B> this Stateflow event input starts the perturbation (triggered on either rising or falling; the Stateflow output event providing this trigger should have its Trigger setting set to ‘either’).  This input will be ignored if the Perturbation block is presently executing a perturbation.
      | <P>
      | <B>reset: </B> this Stateflow event input resets the perturbation (triggered on either rising or falling).  The reset will act immediately and force the Scaling output =0. This does not need to be called between used of the block. If you do not need to stop a perturbation prematurely, then this input can remain unconnected.
      | <P>
      | <B>scaling: </B> this scalar output is the time-dependent window created by this block.  Typically it is wired to the 'scaling' input of another load block.  It ranges in value from 0 to 1.
      | 
      | <H2>Parameters and Dialog Box</H2>
      | <B>Load Table Columns:</B> a 3x1 vector with the elements corresponding to the columns in the Load Table for parameters A, B and C.  If a parameter is not going to be in the Load Table, then the value 0 should be used in the "Load Table Columns" vector (e.g. if there is to be no on-ramp or off-ramp, and the peak-duration coefficients is in column 2, then the "Load Table Columns" vector should be [0 2 0], which indicates that A and C are not specified in the Load Table and so they are set =0).  The same column may be used for more than one parameter, so if the on-ramp and off-ramp are to be equal, then the same column can be specified twice (e.g. [1 2 1]).
      | <P>
      |  All durations are specified in milliseconds.
      | 
      | <H2>Examples</H2>
      | <B>Example 1. </B> Suppose we wish to create a torque pulse with no on or off ramp and a peak duration specified in column 3 of the Load Table.  The 'scaling' output of the Perturbation block would be wired to the 'scaling' input of the Constant_Loads_(joints) block (after setting 'Source for scaling' to 'external' within the Constant_Loads_(joints) block).  The Load Table Columns setting in the dialog box for the Perturbation block would be set to [0 3 0], which indicates no on-ramp or off-ramp and that the peak duration will be in column 3 of the Load Table.
      | <P>
      | <B>Example 2. </B> Suppose we wish to create a force pulse at the hand with an on-ramp and off-ramp of the same duration (specified in column3 of the Load Table) and a peak duration specified in column 4 of the Load Table.  The 'scaling' output of the Perturbation block would be wired to the 'scaling' input of the Constant_Loads_(hand) block (after setting 'Source for scaling' to 'external' within the Constant_Loads_(hand) block).  The Load Table Columns setting in the dialog box for the Perturbation block would be set to [3 4 3], which indicates that the on-ramp and off-ramp durations are specified in column 3 of the Load Table and that the peak duration will be in column 4 of the Load Table.
      | 
      | <H2>Related Blocks </H2>
      | KINARM_Exo_Apply_Loads<BR>
      | Constant_Loads_(hand)<BR>
      | Constant_Loads_(joint)
      mask Callback loadcol:
      | %%%%
      | % Because of bugs iN R2007, R2010a and R2013a (which have been reported to Mathworks), the following code
      | % is required here because in the Initialization Section it will ONLY correctly update those Mask Parameters that are hidden
      | % when the OK button is clicked (NOTE: the initialization code will correctly update all Mask Parameters when the Apply button
      | % is clicked, the bug is that it should also update everything when the OK button is clicked in the absence of an Apply click)
      | %
      | % Adding a set_param call which updates one of the mask parameters will call the initialization code to run, which "avoids"
      | % this bug. This code should be removed once Mathworks has fixed this bug.
      | 
      | temp = get_param(gcb, 'loadcol');
      | set_param(gcb, 'loadcol', temp);
      mask Display:
      | disp(columntext);
      | port_label('output',1,outputname);
      | port_label('input',1, inputname1);
      | port_label('input',2, inputname2);
      | port_label('input',3, inputname3);
  Product : Product  Inputs=3
  Scope 1 : slrtlib/Displays and Logging/Scope   scopeno=4  scopetype=Target  autostart=off  viewmode=Graphical redraw  formatstr='%15.6f'  grid=on  ylimits=[0,0]  nosamples=250  noprepostsamples=0  interleave=1  triggermode=FreeRun  triggersignal=1  trigsignalfromport=off  triggerlevel=0.0  triggerslope=Either  triggerscope=1  triggersample=0  filename=data.dat  mode=Lazy  writesize=512  autorestart=off  dynamicfilemode=off  maxwritefilesize=512*1024^2
  Sum of Elements : Sum  Inputs=+
  Switch : Switch  Criteria=u2 > Threshold
  get fudge factor : Selector  IndexOptions=Index vector (dialog)  Indices=FORCE_MULTIPLIER  OutputSizes=1
  forces (N) : Outport
  wires:
  Compare To Zero1/1 -> Perturbation/2(e_Trigger)
  Sum of Elements/1 -> Compare To Zero1/1
  forces scaling/1 -> Switch/3, Abs/1
  get fudge factor/1 -> Product/1
  Switch/1 -> Memory3/1, Scope 1/1, Product/2
  Perturbation/1(Scaling) -> Product/3, Switch/2
  Abs/1 -> Sum of Elements/1
  Memory3/1 -> Switch/1
  Load Row/1 -> Perturbation/1(Load Row)
  Product/1 -> forces (N)/1
  Task Wide Parameters/1 -> get fudge factor/1

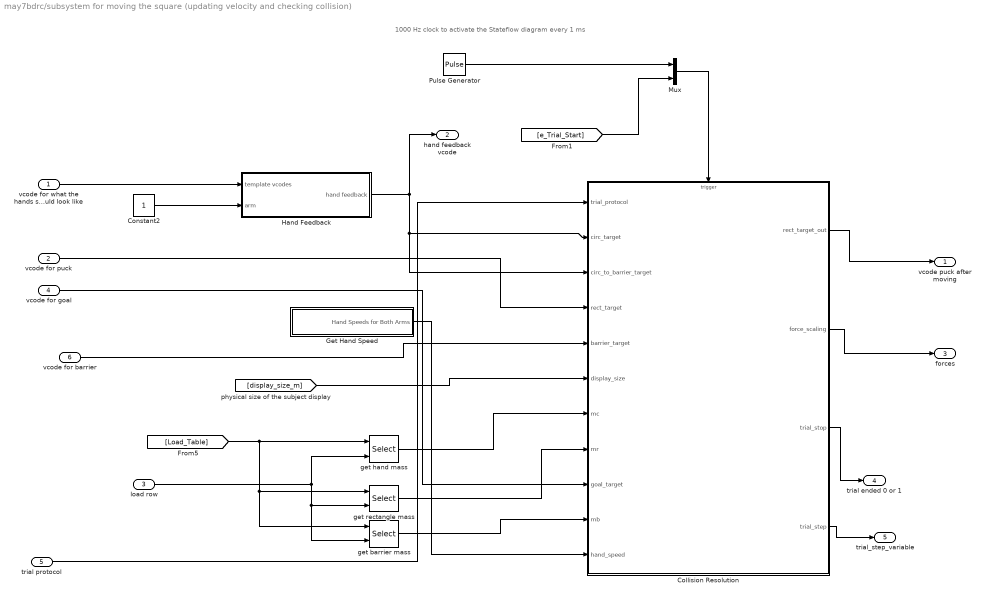
== system may7bdrc/subsystem for moving the square (updating velocity and checking collision) ==
  note: 1000 Hz clock to activate the Stateflow diagram every 1 ms
  vcode for what the hands should look like : Inport  PortDimensions=[1 70]
  vcode for puck : Inport  Port=2  PortDimensions=[1 70]  LockScale=on
  load row : Inport  Port=3
  vcode for goal : Inport  Port=4  PortDimensions=[1 70]
  trial protocol : Inport  Port=5
  vcode for barrier : Inport  Port=6  PortDimensions=[1 70]
  Collision Resolution : Stateflow chart  TreatAsAtomicUnit=on
      settings: PermitHierarchicalResolution=ParametersOnly
  Constant2 : Constant
  Get Hand Speed : Subsystem
  Hand Feedback : Subsystem
  Mux : Mux  Inputs=2
  Pulse Generator : DiscretePulseGenerator  PulseType=Time based  Period=1/1000  PulseWidth=50
  get barrier mass : Selector  NumberOfDimensions=2  IndexOptions=Index vector (port),Index vector (dialog)  Indices=MASS_RECT,MASS_RECT  OutputSizes=1,1
  get hand mass : Selector  NumberOfDimensions=2  IndexOptions=Index vector (port),Index vector (dialog)  Indices=MASS_CIRCLE,MASS_CIRCLE  OutputSizes=1,1
  get rectangle mass : Selector  NumberOfDimensions=2  IndexOptions=Index vector (port),Index vector (dialog)  Indices=MASS_RECT,MASS_RECT  OutputSizes=1,1
  vcode puck after moving : Outport
  hand feedback vcode : Outport  Port=2
  forces : Outport  Port=3
  trial ended 0 or 1 : Outport  Port=4  OutDataTypeStr=double  PortDimensions=[1]
  trial_step_variable : Outport  Port=5  OutDataTypeStr=double  PortDimensions=[1]
  wires:
  load row/1 -> get barrier mass/2, get rectangle mass/2, get hand mass/2
  Hand Feedback/1(hand feedback) -> hand feedback vcode/1, Collision Resolution/3(circ_to_barrier_target), Collision Resolution/2(circ_target)
  Collision Resolution/1(rect_target_out) -> vcode puck after moving/1
  vcode for puck/1 -> Collision Resolution/4(rect_target)
  Get Hand Speed/1(Hand Speeds for Both Arms) -> Collision Resolution/11(hand_speed)
  get hand mass/1 -> Collision Resolution/7(mc)
  get rectangle mass/1 -> Collision Resolution/8(mr)
  Pulse Generator/1 -> Mux/1
  [display_size_m] -> Collision Resolution/6(display_size)
  Collision Resolution/2(force_scaling) -> forces/1
  vcode for what the hands should look like/1 -> Hand Feedback/1(template vcodes)
  Constant2/1 -> Hand Feedback/2(arm)
  Collision Resolution/3(trial_stop) -> trial ended 0 or 1/1
  vcode for goal/1 -> Collision Resolution/9(goal_target)
  trial protocol/1 -> Collision Resolution/1(trial_protocol)
  Collision Resolution/4(trial_step) -> trial_step_variable/1
  vcode for barrier/1 -> Collision Resolution/5(barrier_target)
  [Load_Table] -> get barrier mass/1, get rectangle mass/1, get hand mass/1
  get barrier mass/1 -> Collision Resolution/10(mb)
  [e_Trial_Start] -> Mux/2
  Mux/1 -> Collision Resolution/Trigger
